simulink model "OpenLoopHIL"  (R2025a)
settings: Solver=VariableStepAuto  StartTime=0.0  StopTime=10.0  RelTol=1e-3
undefined symbols (not defined in the file): Down, Pull, w_max
libraries: speedgoatlib_IO691 x3, canmsglib x2, ESys x1, autolibshared x1
settings Model: Creator=tecnicomcbti  LastModifiedBy=tecnicomcbti

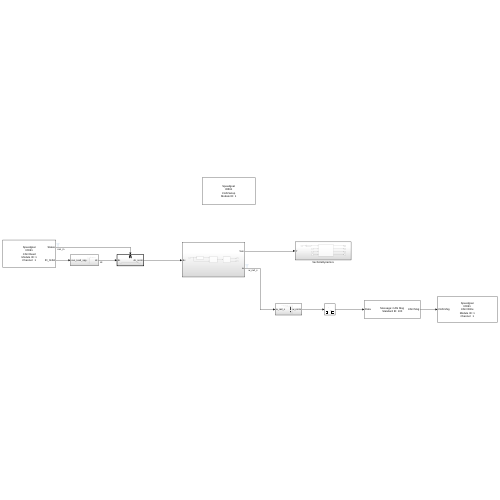
[thumbnail: Simulink's stored preview of the top-level diagram]
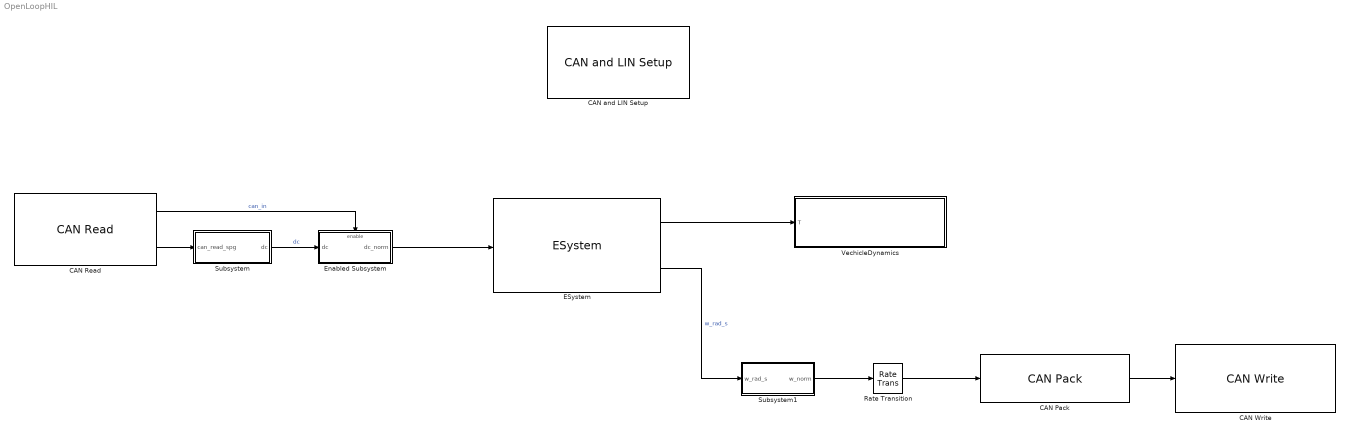
== system OpenLoopHIL ==
  CAN Pack : canmsglib/CAN Pack  MsgList=(none)  MsgName=CAN Msg  MsgIDType=Standard (11-bit identifier)  MsgIdentifier=100  CANIDInput=off  MsgLength=8  Remote=off  ApplyMinMax=off  BusOutput=off  SignalInfo={}
      settings: DataFormat=raw data
  "CAN Read " : speedgoatlib_IO691/CAN Read   moduleType=IO691  id=1  channel=1  messageType=CAN (HS)  useBusOut=off  HasMulRead=Specify by IDs  MsgIDlist=250  isEFF=off  LabelInHex=on  enableInput=off  initValues=[691 1 0.01 0 1 0 0 2 0 1 250]  ts=10e-3
      settings: SourceProductName=IO691
  "CAN Write " : speedgoatlib_IO691/CAN Write   moduleType=IO691  id=1  channel=1  messageType=CAN (HS)  useBusIn=off  numOfMsg=1  enableInput=off  enableStatusPort=off  ts=10e-3  initValues=[691 1 0.01 0 1 0 1 0 0]
      settings: SourceProductName=IO691
  "CAN and LIN Setup " : speedgoatlib_IO691/CAN and LIN Setup   moduleInitValues="[691    1    1   -1   -1]"  id=1  moduleType=IO691  pciSlot=-1  canChn1=CAN (HS)  canChn2=CAN (HS)  canChn3=Disabled  canChn4=Disabled  linChn1=Disabled  linChn2=Disabled  canInitStructArray=[]  canTermStructArray=[]  gpioChnx=Disabled  canChn1InitValues="[2   2   8   1  16   3  19   2   2   5   2   0]"  arbBdrChn1=500 kBaud  clockDividerChn1=Enable  arbManBdrChn1=[8,1,16,3]  fdBdrChn1=5.0 MBaud  fdManBdrChn1=[2,2,5,2]  termResistor1=off  canChn2InitValues="[2   2   8   1  16   3  19   2   2   5   2   0]"  arbBdrChn2=500 kBaud  clockDividerChn2=Enable  arbManBdrChn2=[8,1,16,3]  fdBdrChn2=5.0 MBaud  fdManBdrChn2=[2,2,5,2]  termResistor2=off  canChn3InitValues="[1   0   2   8  31   8  19   2   2   5   2   0]"  arbBdrChn3=1.0 MBaud  clockDividerChn3=Enable  arbManBdrChn3=[2,8,31,8]  fdBdrChn3=5.0 MBaud  fdManBdrChn3=[2,2,5,2]  termResistor3=off  canChn4InitValues="[1   0   2   8  31   8  19   2   2   5   2   0]"  arbBdrChn4=1.0 MBaud  clockDividerChn4=Enable  arbManBdrChn4=[2,8,31,8]  fdBdrChn4=5.0 MBaud  fdManBdrChn4=[2,2,5,2]  termResistor4=off  linChn1InitValues="[0  9600]"  linBtrChn1=9600  linChn2InitValues="[0  9600]"  linBtrChn2=9600  doInitTermStruct="[0  5  0  0  0]"  parDoChannels=[1 2]  parDoVoltage=5  parDoInitValues=0  parDoReset=1  parNumOfDoS=0  parDiChannels=[3 4]  parDiVoltage=5  parDiPull=Pull-Down
      settings: SourceProductName=IO691
  ESystem : ESys/ESystem  SystemSampleTime=-1  VariantActivationTime=update diagram  EmptyChoice=off  PassThrough=off  PassThroughVariantControl=(default)  EmptyChoiceVariantControl=(default)  AllowFlexibleInterface=on  Latency=0  AutoFrameSizeCalculation=off
  Enabled Subsystem : Subsystem  TreatAsAtomicUnit=on
  Rate Transition : RateTransition
  Subsystem : Subsystem
  Subsystem1 : Subsystem
  VechicleDynamics : Subsystem
  wires:
  ESystem/1 -> VechicleDynamics/1(T)
  Subsystem1/1(w_norm) -> Rate Transition/1
  CAN Pack/1 -> "CAN Write "/1
  ESystem/2 -> Subsystem1/1(w_rad_s)  "w_rad_s"
  Rate Transition/1 -> CAN Pack/1
  Enabled Subsystem/1(dc_norm) -> ESystem/1
  "CAN Read "/2 -> Subsystem/1(can_read_spg)
  Subsystem/1(dc) -> Enabled Subsystem/1(dc)  "dc"
  "CAN Read "/1 -> Enabled Subsystem/Enable  "can_in"

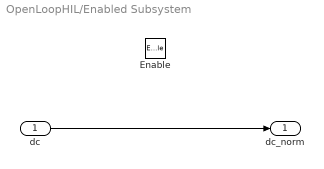
== system OpenLoopHIL/Enabled Subsystem ==
  dc : Inport
  Enable : EnablePort
  dc_norm : Outport
  wires:
  dc/1 -> dc_norm/1

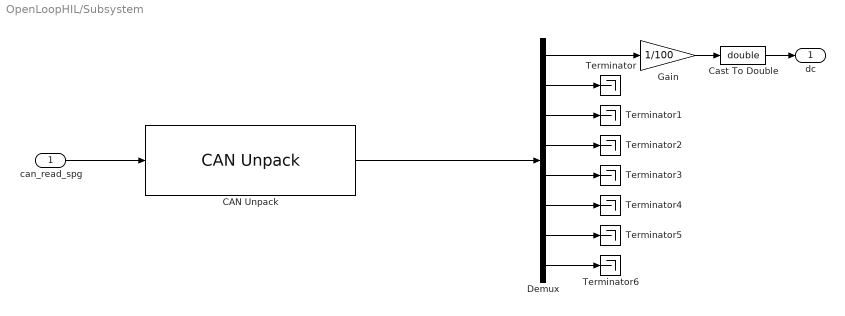
== system OpenLoopHIL/Subsystem ==
  can_read_spg : Inport
  CAN Unpack : canmsglib/CAN Unpack  MsgList=(none)  MsgName=CAN Msg  MsgIDType=Standard (11-bit identifier)  MsgIdentifier=250  MsgLength=8  SignalInfo={}  IDPort=off  TimestampPort=off  ErrorPort=off  RemotePort=off  LengthPort=off  StatusPort=off  ApplyMinMax=off
      settings: DataFormat=raw data
  Cast To Double : DataTypeConversion  OutDataTypeStr=double  SaturateOnIntegerOverflow=off  RndMeth=Floor
  Demux : Demux  Outputs=8
  Gain : Gain  Gain=1/100
  Terminator{,1..6} (7 alike) : Terminator
  dc : Outport
  wires:
  Demux/1 -> Gain/1
  Demux/2 -> Terminator/1
  Demux/3 -> Terminator1/1
  Demux/4 -> Terminator2/1
  Demux/5 -> Terminator3/1
  Demux/6 -> Terminator4/1
  Demux/7 -> Terminator5/1
  Demux/8 -> Terminator6/1
  Cast To Double/1 -> dc/1
  can_read_spg/1 -> CAN Unpack/1
  CAN Unpack/1 -> Demux/1
  Gain/1 -> Cast To Double/1

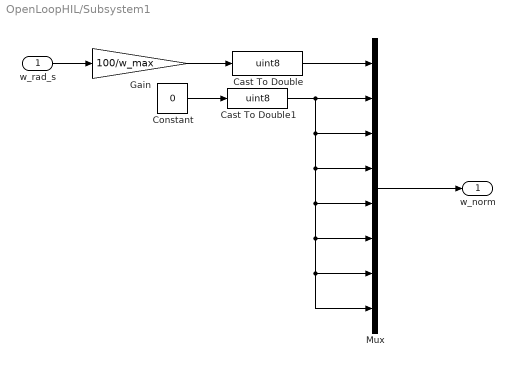
== system OpenLoopHIL/Subsystem1 ==
  w_rad_s : Inport
  Cast To Double : DataTypeConversion  OutDataTypeStr=uint8  SaturateOnIntegerOverflow=off  RndMeth=Floor
  Cast To Double1 : DataTypeConversion  OutDataTypeStr=uint8  SaturateOnIntegerOverflow=off  RndMeth=Floor
  Constant : Constant  Value=0
  Gain : Gain  Gain=100/w_max
  Mux : Mux  Inputs=8
  w_norm : Outport
  wires:
  w_rad_s/1 -> Gain/1
  Cast To Double/1 -> Mux/1
  Constant/1 -> Cast To Double1/1
  Cast To Double1/1 -> Mux/8, Mux/7, Mux/6, Mux/5, Mux/4, Mux/3, Mux/2
  Mux/1 -> w_norm/1
  Gain/1 -> Cast To Double/1

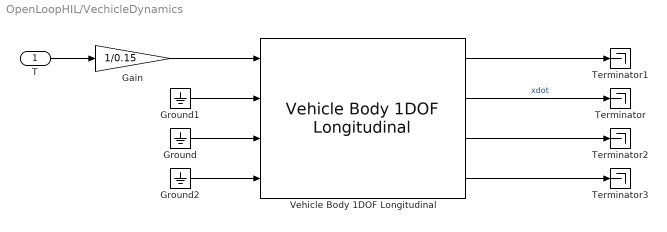
== system OpenLoopHIL/VechicleDynamics ==
  T : Inport
  Gain : Gain  Gain=1/0.15
  Ground : Ground
  Ground1 : Ground
  Ground2 : Ground
  Terminator{,1..3} (4 alike) : Terminator
  Vehicle Body 1DOF Longitudinal : autolibshared/Vehicle Body 1DOF Longitudinal  VariantControl=SL  extFMode=off  extMMode=off  extTamb=off  wind3D=off  aMode=2  NF=2  NR=2  m=50  a=.4  b=.8  h=.6  Cd=.6  Cl=0  Cpm=0  Af=0.15  x_o=0  xdot_o=0  Pabs=101325  T=273  g=9.81
      settings: LibrarySourceBlock=vehdynlibeom/Vehicle Body 1DOF Longitudinal
  wires:
  Gain/1 -> Vehicle Body 1DOF Longitudinal/1
  T/1 -> Gain/1
  Vehicle Body 1DOF Longitudinal/2 -> Terminator/1  "xdot"
  Ground/1 -> Vehicle Body 1DOF Longitudinal/3
  Ground1/1 -> Vehicle Body 1DOF Longitudinal/2
  Ground2/1 -> Vehicle Body 1DOF Longitudinal/4
  Vehicle Body 1DOF Longitudinal/1 -> Terminator1/1
  Vehicle Body 1DOF Longitudinal/3 -> Terminator2/1
  Vehicle Body 1DOF Longitudinal/4 -> Terminator3/1
